simulink model "ThreeWheel_OmniDrive"  (R2018a)
settings: Solver=ode4  StartTime=0.0  StopTime=60  RelTol=1e-3
undefined symbols (not defined in the file): magnitude, tsample
libraries: aerolibutil x2, simulink x2, sharedutil x1
settings Model: Creator=kartik  LastModifiedBy=kartik
settings SolverCC: MaxConsecutiveZCs=100000  ZeroCrossAlgorithm=Adaptive
settings DebuggingCC: MaxConsecutiveZCsMsg=none  IgnoredZcDiagnostic=none

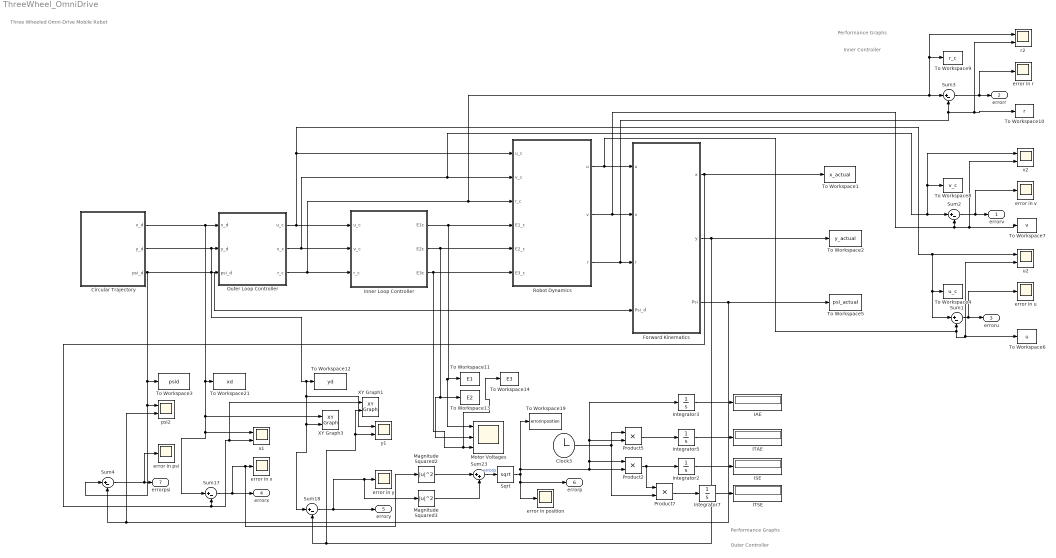
== system ThreeWheel_OmniDrive ==
  note: Three Wheeled Omni-Drive Mobile Robot
  note: Performance Graphs
  note: Inner Controller
  note: Performance Graphs
  note: Outer Controller
  Circular Trajectory : Subsystem  mask{alphae=1, radius=1, radius_final=2, radius_change_time=40, psi_f=.34, psi_change_time=50}
      mask prompts: alphae "Angular velocity of trajectory"; radius "Radius of circle"; radius_final "Final radius of circle"; radius_change_time "Time after change in radius takes place"; psi_f "Final Psi"; psi_change_time "Time after change in Psi takes place"
  Clock3 : Clock
  Forward Kinematics : Subsystem  mask{xi=[0 0 2]}
      mask prompts: xi "Initial Pose [x y psi]"
  IAE : Display
  ISE : Display
  ITAE : Display
  ITSE : Display
  Inner Loop Controller : Subsystem  mask{m=33, Iz=1.35, L=0.25, Ra=0.61, Jo=0.0000097, R=0.06, n=30, K2=0.0292, K3=328, Bo=0.00006, E1max=12, E2max=12, E3max=12}
      mask prompts: m "Mass (in Kg) [m]"; Iz "Inertia of Robot [Iz]"; L "Length between Center of Robot to Wheel (in m) [L]"; Ra "Motor Armature Resistance [Ra]"; Jo "Inertia of Rotor Assembly [Jo]"; R "Wheel Radius [R]"; n "Gear Ratio [n]"; K2 "Motor Torque Constant [K2]"; K3 "Back EMF Constant [K3]"; Bo "Viscous Friction Coefficient of Motor [Bo]"; E1max "Max Voltage of Motor 1 (in V) [E1]"; E2max "Max Voltage of Motor 2 (in V) [E2]"; E3max "Max Voltage of Motor 3 (in V) [E3]"
      mask help: This is the Inner Loop Controller. It produces reference Voltage inputs
  Integrator{2..3,5,7} (4 alike) : Integrator
  Magnitude Squared2 : Math  Operator=magnitude^2  SaturateOnIntegerOverflow=on
  Magnitude Squared3 : Math  Operator=magnitude^2  SaturateOnIntegerOverflow=on
  Motor Voltages : Scope  NumInputPorts=3
  Outer Loop Controller : Subsystem
      mask help: This is the Outer Loop Controller Block. It provides reference velocity signals from the desired trajectory signals. [Inverse Kinematics]
  Product2 : Product
  Product5 : Product
  Product7 : Product
  Robot Dynamics : Subsystem  mask{m=33, Iz=1.35, L=0.25, Ra=0.61, Jo=0.0000097, R=0.06, n=30, K2=0.0292, K3=328, Bo=0.00006, umax=1.18, vmax=1.18, rmax=16.86, dumax=2.5, dvmax=2.5, drmax=2.5}
      mask prompts: m "Mass (in Kg) [m]"; Iz "Inertia of Robot [Iz]"; L "Length between Center of Robot and Wheels (in m) [L]"; Ra "Motor Armature Resistance [Ra]"; Jo "Inertia of Rotor Assembly [Jo]"; R "Wheel Radius [R]"; n "Gear Ratio [n]"; K2 "Motor Torque Constant [K2]"; K3 "Back EMF Constant [K3]"; Bo "Viscous Friction Coefficient of Motor [Bo]"; umax "Maximum Linear Velocity (in m/s) [u]"; vmax "Maximum Linear Velocity(in m/s) [v]"; rmax "Maximum Angular Velocity (in rad/s)"; dumax "Maximum Linear Acceleration (in m/s^2) [du]"; dvmax "Maximum Linear Acceleration(in m/s^2) [dv]"; drmax "Maximum Angular Acceleration (in rad/s^2) [dr]"
      mask help: Dynamics of a 3 wheeled Omni Directional Robot
  Sqrt : Sqrt  SaturateOnIntegerOverflow=on
  Sum{1..4,17..18} (6 alike) : Sum  Inputs=|+-
  Sum23 : Sum  Inputs=|++
  To Workspace1 : ToWorkspace  VariableName=x_actual  SampleTime=-1
  To Workspace10 : ToWorkspace  VariableName=r  SampleTime=-1
  To Workspace11 : ToWorkspace  VariableName=E1  SampleTime=-1
  To Workspace12 : ToWorkspace  VariableName=yd  SampleTime=-1
  To Workspace13 : ToWorkspace  VariableName=E2  SampleTime=-1
  To Workspace14 : ToWorkspace  VariableName=E3  SampleTime=-1
  To Workspace19 : ToWorkspace  VariableName=errorinposition  SampleTime=-1
  To Workspace2 : ToWorkspace  VariableName=y_actual  SampleTime=-1
  To Workspace21 : ToWorkspace  VariableName=xd  SampleTime=-1
  To Workspace3 : ToWorkspace  VariableName=psid  SampleTime=-1
  To Workspace4 : ToWorkspace  VariableName=u_c  SampleTime=-1
  To Workspace5 : ToWorkspace  VariableName=psi_actual  SampleTime=-1
  To Workspace6 : ToWorkspace  VariableName=u  SampleTime=-1
  To Workspace7 : ToWorkspace  VariableName=v  SampleTime=-1
  To Workspace8 : ToWorkspace  VariableName=v_c  SampleTime=-1
  To Workspace9 : ToWorkspace  VariableName=r_c  SampleTime=-1
  XY Graph1 : simulink/Sinks/XY Graph  xmin=-4  xmax=4  ymin=-4  ymax=4  st=.1
  XY Graph3 : simulink/Sinks/XY Graph  xmin=-4  xmax=4  ymin=-4  ymax=4  st=.1
  error in position : Scope
  error in psi : Scope
  error in r : Scope
  error in u : Scope
  error in v : Scope
  error in x : Scope
  error in y : Scope
  psi2 : Scope  NumInputPorts=2
  r2 : Scope  NumInputPorts=2
  u2 : Scope  NumInputPorts=2
  v2 : Scope  NumInputPorts=2
  x1 : Scope  NumInputPorts=2
  y1 : Scope  NumInputPorts=2
  errorv : Outport
  errorr : Outport  Port=2
  erroru : Outport  Port=3
  errorx : Outport  Port=4
  errory : Outport  Port=5
  errorp : Outport  Port=6
  errorpsi : Outport  Port=7
  wires:
  Outer Loop Controller/1(u_c) -> Sum1/1, To Workspace4/1, u2/1, Robot Dynamics/1(u_c), Inner Loop Controller/1(u_c)
  Outer Loop Controller/2(v_c) -> Robot Dynamics/2(v_c), v2/1, To Workspace8/1, Sum2/1, Inner Loop Controller/2(v_c)
  Outer Loop Controller/3(r_c) -> r2/1, To Workspace9/1, Sum3/1, Robot Dynamics/3(r_c), Inner Loop Controller/3(r_c)
  Inner Loop Controller/3(E3c) -> To Workspace14/1, Motor Voltages/3, Robot Dynamics/6(E3_c)
  Inner Loop Controller/2(E2c) -> Motor Voltages/2, To Workspace13/1, Robot Dynamics/5(E2_c)
  Inner Loop Controller/1("E1c ") -> Motor Voltages/1, To Workspace11/1, Robot Dynamics/4(E1_c)
  Robot Dynamics/3(r) -> To Workspace10/1, r2/2, Sum3/2, Forward Kinematics/3(r)
  Robot Dynamics/2(v) -> Forward Kinematics/2(v), To Workspace7/1, v2/2, Sum2/2
  Robot Dynamics/1("u ") -> To Workspace6/1, u2/2, Sum1/2, Forward Kinematics/1(u)
  Forward Kinematics/3(Psi) -> psi2/2, Sum4/2, To Workspace5/1
  Sum1/1 -> error in u/1, erroru/1
  Forward Kinematics/1(x) -> XY Graph1/1, x1/2, Sum17/2, To Workspace1/1
  Product2/1 -> Integrator2/1, Product7/1
  Magnitude Squared2/1 -> Sum23/1
  Forward Kinematics/2(y) -> XY Graph1/2, y1/2, Sum18/2, To Workspace2/1
  Sum18/1 -> Magnitude Squared3/1, error in y/1, errory/1
  Integrator3/1 -> IAE/1
  Integrator7/1 -> ITSE/1
  Sum23/1 -> Sqrt/1  "errorp"
  Clock3/1 -> Product5/1, Product7/2
  Product7/1 -> Integrator7/1
  Integrator5/1 -> ITAE/1
  Sum17/1 -> errorx/1, Magnitude Squared2/1, error in x/1
  Magnitude Squared3/1 -> Sum23/2
  Product5/1 -> Integrator5/1
  Sqrt/1 -> To Workspace19/1, Product2/2, Product2/1, Product5/2, Integrator3/1, errorp/1, error in position/1
  Integrator2/1 -> ISE/1
  Sum2/1 -> error in v/1, errorv/1
  Sum3/1 -> error in r/1, errorr/1
  Sum4/1 -> error in psi/1, errorpsi/1
  Circular Trajectory/2(y_d) -> y1/1, Sum18/1, XY Graph3/2, To Workspace12/1, Outer Loop Controller/2(y_d)
  Circular Trajectory/3(psi_d) -> psi2/1, Sum4/1, To Workspace3/1, Forward Kinematics/4(Psi_d), Outer Loop Controller/3(psi_d)
  Circular Trajectory/1(x_d) -> XY Graph3/1, Sum17/1, x1/1, To Workspace21/1, Outer Loop Controller/1(x_d)

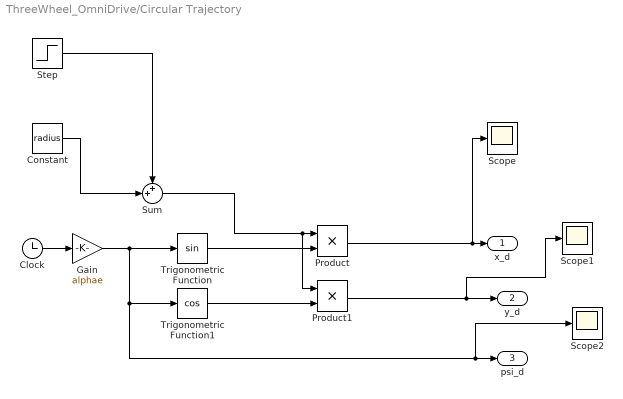
== system ThreeWheel_OmniDrive/Circular Trajectory ==
  Clock : Clock
  Constant : Constant  Value=radius
  Gain : Gain  Gain=alphae
  Product : Product
  Product1 : Product
  Scope : Scope
  Scope1 : Scope
  Scope2 : Scope
  Step : Step  Time=radius_change_time  After=radius_final  SampleTime=0
  Sum : Sum  Inputs=++|
  Trigonometric Function : Trigonometry
  Trigonometric Function1 : Trigonometry  Operator=cos
  x_d : Outport
  y_d : Outport  Port=2
  psi_d : Outport  Port=3
  wires:
  Sum/1 -> Product1/1, Product/1
  Clock/1 -> Gain/1
  Trigonometric Function1/1 -> Product1/2
  Constant/1 -> Sum/2
  Step/1 -> Sum/1
  Gain/1 -> Trigonometric Function/1, Scope2/1, psi_d/1, Trigonometric Function1/1
  Trigonometric Function/1 -> Product/2
  Product1/1 -> Scope1/1, y_d/1
  Product/1 -> Scope/1, x_d/1

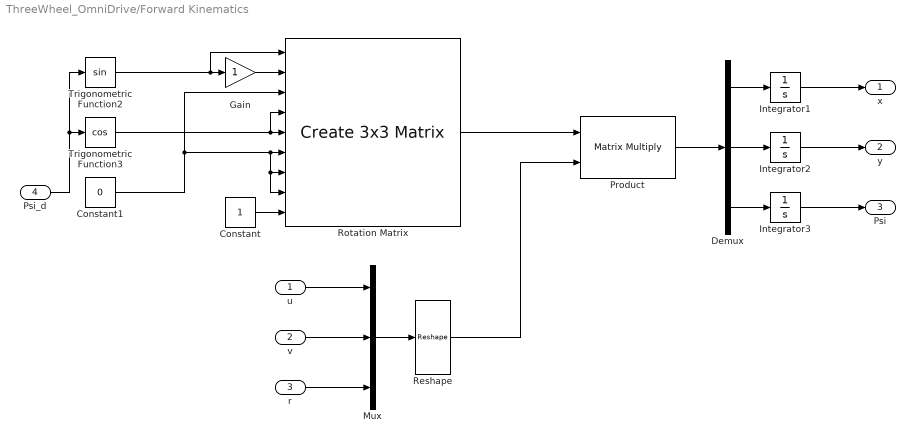
== system ThreeWheel_OmniDrive/Forward Kinematics ==
  u : Inport
  v : Inport  Port=2
  r : Inport  Port=3
  Psi_d : Inport  Port=4
  Constant : Constant  SampleTime=tsample
  Constant1 : Constant  Value=0  SampleTime=tsample
  Demux : Demux  Outputs=3
  Gain : Gain
  Integrator1 : Integrator  InitialCondition=xi(1)
  Integrator2 : Integrator  InitialCondition=xi(2)
  Integrator3 : Integrator  InitialCondition=xi(3)
  Mux : Mux  Inputs=3
  Product : Product  Multiplication=Matrix(*)
  Reshape : Reshape  OutputDimensionality=Column vector (2-D)
  Rotation Matrix : sharedutil/Create 3x3 Matrix  aMode=aMode
  Trigonometric Function2 : Trigonometry
  Trigonometric Function3 : Trigonometry  Operator=cos
  x : Outport
  y : Outport  Port=2
  Psi : Outport  Port=3
  wires:
  Trigonometric Function3/1 -> Rotation Matrix/4, Rotation Matrix/5
  Trigonometric Function2/1 -> Rotation Matrix/1, Gain/1
  Constant1/1 -> Rotation Matrix/3, Rotation Matrix/8, Rotation Matrix/7, Rotation Matrix/6
  Integrator3/1 -> Psi/1
  Psi_d/1 -> Trigonometric Function2/1, Trigonometric Function3/1
  v/1 -> Mux/2
  Demux/2 -> Integrator2/1
  Demux/1 -> Integrator1/1
  Product/1 -> Demux/1
  Gain/1 -> Rotation Matrix/2
  Constant/1 -> Rotation Matrix/9
  Demux/3 -> Integrator3/1
  Integrator1/1 -> x/1
  Rotation Matrix/1 -> Product/1
  Reshape/1 -> Product/2
  r/1 -> Mux/3
  Mux/1 -> Reshape/1
  u/1 -> Mux/1
  Integrator2/1 -> y/1

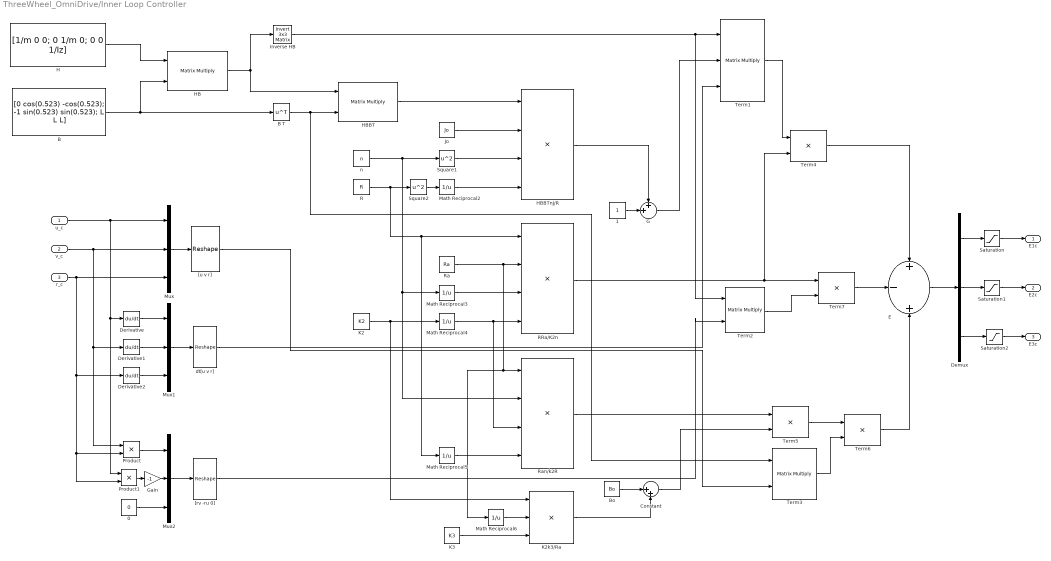
== system ThreeWheel_OmniDrive/Inner Loop Controller ==
  u_c : Inport
  v_c : Inport  Port=2
  r_c : Inport  Port=3
  "0 " : Constant  Value=0  SampleTime=tsample
  1 : Constant  SampleTime=tsample
  B : Constant  Value=[0 cos(0.523) -cos(0.523); -1 sin(0.523) sin(0.523); L L L]  SampleTime=tsample
  B T : Math  Operator=transpose  SaturateOnIntegerOverflow=on
  Bo : Constant  Value=Bo  SampleTime=tsample
  Constant : Sum  Inputs=|++
  Demux : Demux  Outputs=3
  Derivative : Derivative
  Derivative1 : Derivative
  Derivative2 : Derivative
  E : Sum  Inputs=+-+
  G : Sum  Inputs=++|
  Gain : Gain  Gain=-1
  H : Constant  Value=[1/m 0 0; 0 1/m 0; 0 0 1/Iz]  SampleTime=tsample
  HB : Product  Multiplication=Matrix(*)
  HBBT : Product  Multiplication=Matrix(*)
  HBBTnJ/R : Product  Inputs=4
  Inverse HB : aerolibutil/Invert  3x3 Matrix
  Jo : Constant  Value=Jo  SampleTime=tsample
  K2 : Constant  Value=K2  SampleTime=tsample
  K2k3/Ra : Product  Inputs=3
  K3 : Constant  Value=K3  SampleTime=tsample
  Math Reciprocal{2..6} (5 alike) : Math  Operator=reciprocal  SaturateOnIntegerOverflow=on
  Mux : Mux  Inputs=3
  Mux1 : Mux  Inputs=3
  Mux2 : Mux  Inputs=3
  Product : Product
  Product1 : Product
  R : Constant  Value=R  SampleTime=tsample
  RRa/K2n : Product  Inputs=4
  Ra : Constant  Value=Ra  SampleTime=tsample
  Ran/k2R : Product  Inputs=4
  Saturation : Saturate  UpperLimit=E1max  LowerLimit=-E1max
  Saturation1 : Saturate  UpperLimit=E2max  LowerLimit=-E2max
  Saturation2 : Saturate  UpperLimit=E3max  LowerLimit=-E3max
  Square1 : Math  Operator=square  SaturateOnIntegerOverflow=on
  Square2 : Math  Operator=square  SaturateOnIntegerOverflow=on
  Term1 : Product  Inputs=3  Multiplication=Matrix(*)
  Term2 : Product  Multiplication=Matrix(*)
  Term3 : Product  Multiplication=Matrix(*)
  Term{4..7} (4 alike) : Product
  "[rv -ru 0]" : Reshape  OutputDimensionality=Column vector (2-D)  OutputDimensions=[3,1]
  "[u v r]" : Reshape  OutputDimensionality=Column vector (2-D)  OutputDimensions=[3,1]
  dt[u v r] : Reshape  OutputDimensionality=Column vector (2-D)  OutputDimensions=[3,1]
  n : Constant  Value=n  SampleTime=tsample
  "E1c " : Outport
  E2c : Outport  Port=2
  E3c : Outport  Port=3
  wires:
  R/1 -> RRa/K2n/1, Math Reciprocal5/1, Square2/1
  RRa/K2n/1 -> Term7/1, Term4/2
  K2/1 -> K2k3/Ra/1, Math Reciprocal4/1
  Ra/1 -> Ran/k2R/1, Math Reciprocal6/1, RRa/K2n/2
  v_c/1 -> Mux/2, Derivative1/1, Product/1
  HB/1 -> HBBT/1, Inverse HB/1
  Square1/1 -> HBBTnJ/R/3
  Derivative/1 -> Mux1/1
  Math Reciprocal6/1 -> K2k3/Ra/2
  r_c/1 -> Mux/3, Derivative2/1, Product/2, Product1/2
  Math Reciprocal4/1 -> RRa/K2n/4, Ran/k2R/3
  K2k3/Ra/1 -> Constant/2
  B/1 -> HB/2, B T/1
  B T/1 -> Term3/1, HBBT/2
  Mux1/1 -> dt[u v r]/1
  n/1 -> Math Reciprocal3/1, Ran/k2R/2, Square1/1
  Inverse HB/1 -> Term1/1, Term2/1
  HBBTnJ/R/1 -> G/1
  Bo/1 -> Constant/1
  Math Reciprocal3/1 -> RRa/K2n/3
  Derivative2/1 -> Mux1/3
  Mux/1 -> "[u v r]"/1
  Square2/1 -> Math Reciprocal2/1
  Product/1 -> Mux2/1
  u_c/1 -> Mux/1, Derivative/1, Product1/1
  Gain/1 -> Mux2/2
  Math Reciprocal5/1 -> Ran/k2R/4
  Product1/1 -> Gain/1
  Constant/1 -> Term5/2
  HBBT/1 -> HBBTnJ/R/1
  1/1 -> G/2
  K3/1 -> K2k3/Ra/3
  Jo/1 -> HBBTnJ/R/2
  Mux2/1 -> "[rv -ru 0]"/1
  Derivative1/1 -> Mux1/2
  H/1 -> HB/1
  "0 "/1 -> Mux2/3
  Math Reciprocal2/1 -> HBBTnJ/R/4
  "[u v r]"/1 -> Term3/2
  dt[u v r]/1 -> Term1/3
  "[rv -ru 0]"/1 -> Term2/2
  Term1/1 -> Term4/1
  Term4/1 -> E/1
  G/1 -> Term1/2
  Term3/1 -> Term6/2
  Ran/k2R/1 -> Term5/1
  Term5/1 -> Term6/1
  Term6/1 -> E/3
  Term7/1 -> E/2
  Term2/1 -> Term7/2
  E/1 -> Demux/1
  Demux/1 -> Saturation/1
  Demux/2 -> Saturation1/1
  Demux/3 -> Saturation2/1
  Saturation/1 -> "E1c "/1
  Saturation2/1 -> E3c/1
  Saturation1/1 -> E2c/1

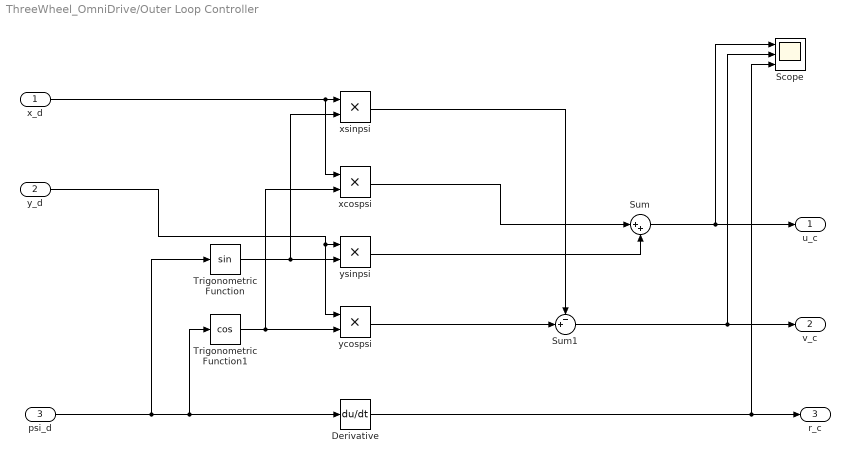
== system ThreeWheel_OmniDrive/Outer Loop Controller ==
  x_d : Inport
  y_d : Inport  Port=2
  psi_d : Inport  Port=3
  Derivative : Derivative
  Scope : Scope  NumInputPorts=3
  Sum : Sum  Inputs=|++
  Sum1 : Sum  Inputs=-+|
  Trigonometric Function : Trigonometry
  Trigonometric Function1 : Trigonometry  Operator=cos
  xcospsi : Product
  xsinpsi : Product
  ycospsi : Product
  ysinpsi : Product
  u_c : Outport
  v_c : Outport  Port=2
  r_c : Outport  Port=3
  wires:
  Sum/1 -> Scope/1, u_c/1
  ysinpsi/1 -> Sum/2
  Trigonometric Function1/1 -> ycospsi/2, xcospsi/2
  Trigonometric Function/1 -> ysinpsi/2, xsinpsi/2
  Derivative/1 -> Scope/3, r_c/1
  x_d/1 -> xcospsi/1, xsinpsi/1
  psi_d/1 -> Trigonometric Function/1, Trigonometric Function1/1, Derivative/1
  ycospsi/1 -> Sum1/2
  xcospsi/1 -> Sum/1
  y_d/1 -> ycospsi/1, ysinpsi/1
  Sum1/1 -> Scope/2, v_c/1
  xsinpsi/1 -> Sum1/1

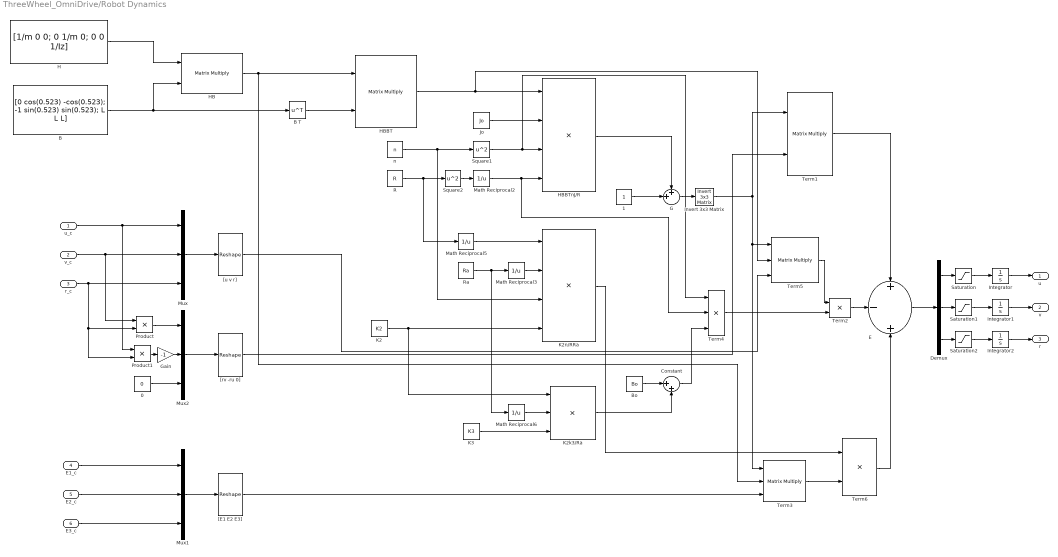
== system ThreeWheel_OmniDrive/Robot Dynamics ==
  u_c : Inport
  v_c : Inport  Port=2
  r_c : Inport  Port=3
  E1_c : Inport  Port=4
  E2_c : Inport  Port=5
  E3_c : Inport  Port=6
  "0 " : Constant  Value=0  SampleTime=tsample
  1 : Constant  SampleTime=tsample
  B : Constant  Value=[0 cos(0.523) -cos(0.523); -1 sin(0.523) sin(0.523); L L L]  SampleTime=tsample
  B T : Math  Operator=transpose  SaturateOnIntegerOverflow=on
  Bo : Constant  Value=Bo  SampleTime=tsample
  Constant : Sum  Inputs=|++
  Demux : Demux  Outputs=3
  E : Sum  Inputs=+-+
  G : Sum  Inputs=++|
  Gain : Gain  Gain=-1
  H : Constant  Value=[1/m 0 0; 0 1/m 0; 0 0 1/Iz]  SampleTime=tsample
  HB : Product  Multiplication=Matrix(*)
  HBBT : Product  Multiplication=Matrix(*)
  HBBTnJ/R : Product  Inputs=4
  Integrator : Integrator  LimitOutput=on  UpperSaturationLimit=umax  LowerSaturationLimit=-umax
  Integrator1 : Integrator  LimitOutput=on  UpperSaturationLimit=vmax  LowerSaturationLimit=-vmax
  Integrator2 : Integrator  LimitOutput=on  UpperSaturationLimit=rmax  LowerSaturationLimit=-rmax
  Invert 3x3 Matrix : aerolibutil/Invert  3x3 Matrix
  Jo : Constant  Value=Jo  SampleTime=tsample
  K2 : Constant  Value=K2  SampleTime=tsample
  K2k3/Ra : Product  Inputs=3
  K2n/RRa : Product  Inputs=4
  K3 : Constant  Value=K3  SampleTime=tsample
  Math Reciprocal{2..3,5..6} (4 alike) : Math  Operator=reciprocal  SaturateOnIntegerOverflow=on
  Mux : Mux  Inputs=3
  Mux1 : Mux  Inputs=3
  Mux2 : Mux  Inputs=3
  Product : Product
  Product1 : Product
  R : Constant  Value=R  SampleTime=tsample
  Ra : Constant  Value=Ra  SampleTime=tsample
  Saturation : Saturate  UpperLimit=dumax  LowerLimit=-dumax
  Saturation1 : Saturate  UpperLimit=dvmax  LowerLimit=-dvmax
  Saturation2 : Saturate  UpperLimit=drmax  LowerLimit=-drmax
  Square1 : Math  Operator=square  SaturateOnIntegerOverflow=on
  Square2 : Math  Operator=square  SaturateOnIntegerOverflow=on
  Term1 : Product  Multiplication=Matrix(*)
  Term2 : Product
  Term3 : Product  Inputs=3  Multiplication=Matrix(*)
  Term4 : Product  Inputs=3
  Term5 : Product  Inputs=3  Multiplication=Matrix(*)
  Term6 : Product
  "[E1 E2 E3]" : Reshape  OutputDimensionality=Column vector (2-D)  OutputDimensions=[3,1]
  "[rv -ru 0]" : Reshape  OutputDimensionality=Column vector (2-D)  OutputDimensions=[3,1]
  "[u v r]" : Reshape  OutputDimensionality=Column vector (2-D)  OutputDimensions=[3,1]
  n : Constant  Value=n  SampleTime=tsample
  "u " : Outport
  v : Outport  Port=2
  r : Outport  Port=3
  wires:
  Demux/3 -> Saturation2/1
  Demux/1 -> Saturation/1
  G/1 -> Invert 3x3 Matrix/1
  Invert 3x3 Matrix/1 -> Term3/1, Term5/1, Term1/1
  v_c/1 -> Mux/2, Product/1
  K2/1 -> K2n/RRa/4, K2k3/Ra/1
  Product/1 -> Mux2/1
  K2k3/Ra/1 -> Constant/2
  n/1 -> K2n/RRa/3, Square1/1
  Mux2/1 -> "[rv -ru 0]"/1
  B T/1 -> HBBT/2
  Jo/1 -> HBBTnJ/R/2
  Demux/2 -> Saturation1/1
  E3_c/1 -> Mux1/3
  Square1/1 -> Term4/1, HBBTnJ/R/3
  B/1 -> HB/2, B T/1
  Math Reciprocal5/1 -> K2n/RRa/1
  E1_c/1 -> Mux1/1
  u_c/1 -> Mux/1, Product1/1
  r_c/1 -> Mux/3, Product/2, Product1/2
  Term1/1 -> E/1
  HB/1 -> Term3/2, HBBT/1
  K3/1 -> K2k3/Ra/3
  Math Reciprocal2/1 -> Term4/2, HBBTnJ/R/4
  1/1 -> G/2
  Math Reciprocal6/1 -> K2k3/Ra/2
  "0 "/1 -> Mux2/3
  H/1 -> HB/1
  Mux/1 -> "[u v r]"/1
  "[rv -ru 0]"/1 -> Term1/2
  HBBT/1 -> Term5/2, HBBTnJ/R/1
  Gain/1 -> Mux2/2
  E/1 -> Demux/1
  Square2/1 -> Math Reciprocal2/1
  Product1/1 -> Gain/1
  "[E1 E2 E3]"/1 -> Term3/3
  R/1 -> Math Reciprocal5/1, Square2/1
  Term2/1 -> E/2
  Integrator1/1 -> v/1
  Term6/1 -> E/3
  Math Reciprocal3/1 -> K2n/RRa/2
  K2n/RRa/1 -> Term6/1
  HBBTnJ/R/1 -> G/1
  Bo/1 -> Constant/1
  E2_c/1 -> Mux1/2
  Integrator/1 -> "u "/1
  Integrator2/1 -> r/1
  Ra/1 -> Math Reciprocal3/1, Math Reciprocal6/1
  Mux1/1 -> "[E1 E2 E3]"/1
  "[u v r]"/1 -> Term5/3
  Constant/1 -> Term4/3
  Term4/1 -> Term2/2
  Term5/1 -> Term2/1
  Term3/1 -> Term6/2
  Saturation/1 -> Integrator/1
  Saturation1/1 -> Integrator1/1
  Saturation2/1 -> Integrator2/1
